simulink model "GATOUP"  (R2022b)
settings: configuration reference "SharedConfig" (kept outside this file)
values from neighbouring files (symbols this model uses):
  PhaAPwmDcDialEna_C = 0.0    [GATOUP.sldd]
  PhaAPwmDcDialVal_C = 1000.0    [GATOUP.sldd]
  PhaBPwmDcDialEna_C = 0.0    [GATOUP.sldd]
  PhaBPwmDcDialVal_C = 1000.0    [GATOUP.sldd]
  PhaCPwmDcDialEna_C = 0.0    [GATOUP.sldd]
  PhaCPwmDcDialVal_C = 600.0    [GATOUP.sldd]
  ReloadRegisterMax_C = 12000.0    [GATOUP.sldd]
undefined symbols (not defined in the file or in its folder): slcm
libraries: simulink x1
Description:
  | Converts phase voltage commands into phase modulation commands.
settings Model: DataDictionary=GATOUP.sldd  Creator=Kevin  LastModifiedBy=Max Kolesnikov
settings ConfigSetRef: SourceName=SharedConfig

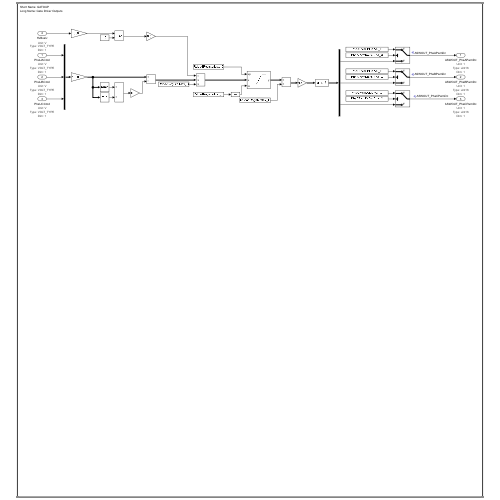
[thumbnail: Simulink's stored preview of the top-level diagram]
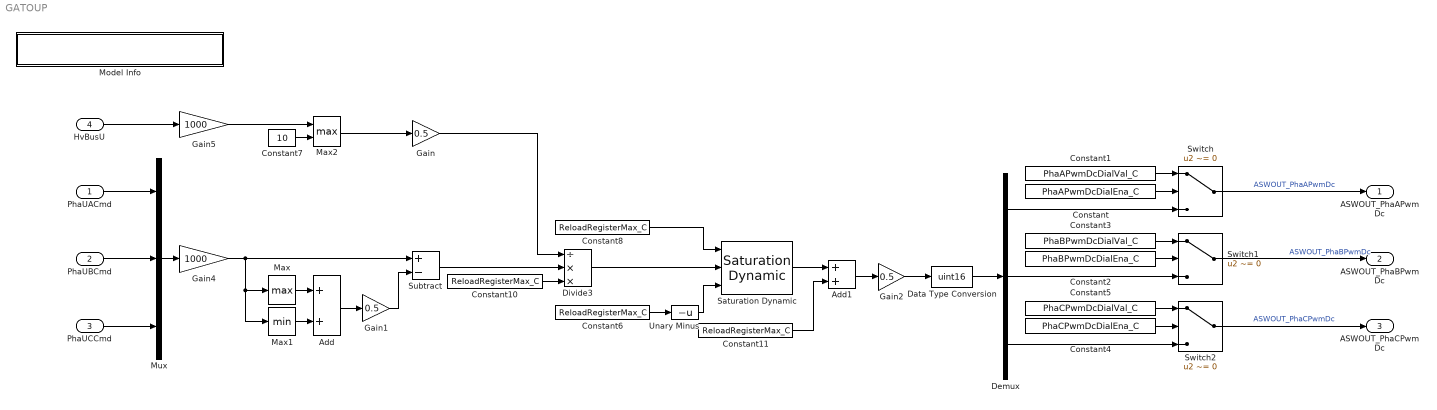
== system GATOUP ==
  PhaUACmd : Inport  OutDataTypeStr=VOLT_TYPE  Unit=V  PortDimensions=1
      settings: AttributesFormatString=|
      | Unit: %<Unit>
      | Type: %<OutDataTypeStr>
      | Dim: %<PortDimensions>
  PhaUBCmd : Inport  Port=2  OutDataTypeStr=VOLT_TYPE  Unit=V  PortDimensions=1
      settings: AttributesFormatString=|
      | Unit: %<Unit>
      | Type: %<OutDataTypeStr>
      | Dim: %<PortDimensions>
  PhaUCCmd : Inport  Port=3  OutDataTypeStr=VOLT_TYPE  Unit=V  PortDimensions=1
      settings: AttributesFormatString=|
      | Unit: %<Unit>
      | Type: %<OutDataTypeStr>
      | Dim: %<PortDimensions>
  HvBusU : Inport  Port=4  OutDataTypeStr=VOLT_TYPE  Unit=V  PortDimensions=1
      settings: AttributesFormatString=|
      | Unit: %<Unit>
      | Type: %<OutDataTypeStr>
      | Dim: %<PortDimensions>
  Add : Sum
  Add1 : Sum
  Constant : Constant  Value=PhaAPwmDcDialEna_C
  Constant1 : Constant  Value=PhaAPwmDcDialVal_C
  Constant{6,8,10..11} (4 alike) : Constant  Value=ReloadRegisterMax_C
  Constant2 : Constant  Value=PhaBPwmDcDialEna_C
  Constant3 : Constant  Value=PhaBPwmDcDialVal_C
  Constant4 : Constant  Value=PhaCPwmDcDialEna_C
  Constant5 : Constant  Value=PhaCPwmDcDialVal_C
  Constant7 : Constant  Value=10  OutDataTypeStr=VOLT_TYPE
  Data Type Conversion : DataTypeConversion  OutDataTypeStr=uint16  SaturateOnIntegerOverflow=off  RndMeth=Floor
  Demux : Demux  Outputs=3
  Divide3 : Product  Inputs=/**  OutDataTypeStr=int16
  Gain : Gain  Gain=0.5  OutDataTypeStr=Inherit: Same as input  ParamDataTypeStr=Inherit: Same as input
  Gain1 : Gain  Gain=0.5  OutDataTypeStr=Inherit: Same as input  ParamDataTypeStr=Inherit: Same as input
  Gain2 : Gain  Gain=0.5  OutDataTypeStr=int16
  Gain4 : Gain  Gain=1000  OutDataTypeStr=Inherit: Same as input  ParamDataTypeStr=Inherit: Same as input
  Gain5 : Gain  Gain=1000  OutDataTypeStr=Inherit: Same as input  ParamDataTypeStr=Inherit: Same as input
  Max : MinMax  Function=max
  Max1 : MinMax
  Max2 : MinMax  Function=max  Inputs=2
  Model Info : Subsystem  LoadFcn=slcm LoadBlock;  InitFcn=slcm('UpdateAllCMBlocksInThisModelInit')  mask(CMBlock){Frame=off, DisplayStringWithTags=|, MaskDisplayString=Short Name: GATOUP\nLong Name: Gate Driver Outputs, HorizontalTextAlignment=Left, LeftAlignmentValue=0.02}
      mask DisplayStringWithTags=|
      | Short Name: %<ModelName>
      | Long Name: Gate Driver Outputs
      mask prompts: Frame "Simulink:masks:Frame_MP"; DisplayStringWithTags "Simulink:masks:DisplayStringWithTags_MP"; MaskDisplayString "Simulink:masks:MaskDisplayString_MP"; HorizontalTextAlignment "Simulink:masks:HorizontalTextAlignment_MP"; LeftAlignmentValue "Simulink:masks:LeftAlignmentValue_MP"
      mask help: Simulink:masks:CMBlock_MD
      settings: CopyFcn=slcm CopyBlock;  DeleteFcn=slcm Cancel;  PostSaveFcn=slcm('UpdateAllCMBlocksInThisModel')  NameChangeFcn=slcm Rename;  OpenFcn=slcm
      mask Display: text(slResolve(LeftAlignmentValue, gcbh), 0.5, MaskDisplayString, 'HorizontalAlignment', HorizontalTextAlignment)
  Mux : Mux  Inputs=3
  Saturation Dynamic : simulink/Discontinuities/Saturation Dynamic  OutMin=[]  OutMax=[]  OutDataTypeStr=Inherit: Same as second input  OutDataType=fixdt(1, 16)  OutScaling=2^-10  DoSatur=off
  Subtract : Sum  Inputs=+-
  Switch : Switch  Criteria=u2 ~= 0  SaturateOnIntegerOverflow=off  InputSameDT=off
  Switch1 : Switch  Criteria=u2 ~= 0  SaturateOnIntegerOverflow=off  InputSameDT=off
  Switch2 : Switch  Criteria=u2 ~= 0  SaturateOnIntegerOverflow=off  InputSameDT=off
  Unary Minus : UnaryMinus
  ASWOUT_PhaAPwmDc : Outport  OutDataTypeStr=uint16  Unit=1  PortDimensions=1
      settings: AttributesFormatString=|
      | Unit: %<Unit>
      | Type: %<OutDataTypeStr>
      | Dim: %<PortDimensions>
  ASWOUT_PhaBPwmDc : Outport  Port=2  OutDataTypeStr=uint16  Unit=1  PortDimensions=1
      settings: AttributesFormatString=|
      | Unit: %<Unit>
      | Type: %<OutDataTypeStr>
      | Dim: %<PortDimensions>
  ASWOUT_PhaCPwmDc : Outport  Port=3  OutDataTypeStr=uint16  Unit=1  PortDimensions=1
      settings: AttributesFormatString=|
      | Unit: %<Unit>
      | Type: %<OutDataTypeStr>
      | Dim: %<PortDimensions>
  wires:
  Switch/1 -> ASWOUT_PhaAPwmDc/1  "ASWOUT_PhaAPwmDc"
  Constant/1 -> Switch/2
  Constant1/1 -> Switch/1
  Constant3/1 -> Switch1/1
  Constant2/1 -> Switch1/2
  Switch1/1 -> ASWOUT_PhaBPwmDc/1  "ASWOUT_PhaBPwmDc"
  Switch2/1 -> ASWOUT_PhaCPwmDc/1  "ASWOUT_PhaCPwmDc"
  Constant4/1 -> Switch2/2
  Constant5/1 -> Switch2/1
  Max/1 -> Add/1
  Max1/1 -> Add/2
  Subtract/1 -> Divide3/2
  Gain1/1 -> Subtract/2
  Gain/1 -> Divide3/1
  Mux/1 -> Gain4/1
  Add/1 -> Gain1/1
  PhaUCCmd/1 -> Mux/3
  PhaUBCmd/1 -> Mux/2
  PhaUACmd/1 -> Mux/1
  HvBusU/1 -> Gain5/1
  Divide3/1 -> Saturation Dynamic/2
  Saturation Dynamic/1 -> Add1/1
  Demux/1 -> Switch/3
  Demux/2 -> Switch1/3
  Demux/3 -> Switch2/3
  Add1/1 -> Gain2/1
  Data Type Conversion/1 -> Demux/1
  Max2/1 -> Gain/1
  Constant7/1 -> Max2/2
  Gain4/1 -> Max1/1, Max/1, Subtract/1
  Gain5/1 -> Max2/1
  Gain2/1 -> Data Type Conversion/1
  Constant10/1 -> Divide3/3
  Constant11/1 -> Add1/2
  Constant6/1 -> Unary Minus/1
  Unary Minus/1 -> Saturation Dynamic/3
  Constant8/1 -> Saturation Dynamic/1

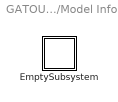
== system GATOUP/Model Info ==
  EmptySubsystem : Subsystem

== system GATOUP/Model Info/EmptySubsystem ==
